simulink model "PIDp2"  (R2016b)
settings: Solver=FixedStepAuto  StartTime=0.0  StopTime=10.0  FixedStep=0.01  RelTol=1e-3
values from neighbouring files (symbols this model uses):
  den = [1 0.1313 1.109]    [UpdatedSimulinkValues-2.m]    (also in UpdatedSimulinkValuesalex1.m; part2a.m)
  Kd = G    [UpdatedSimulinkValues-2.m]    (also in UpdatedSimulinkValuesalex1.m; part2a.m = 0.1)
  Ki = G    [UpdatedSimulinkValues-2.m]    (also in UpdatedSimulinkValuesalex1.m; part2a.m = 0.1)
  Kp = G    [UpdatedSimulinkValues-2.m]    (also in UpdatedSimulinkValuesalex1.m; part2a.m = 0.1)
  num = [0.26*1.109*180/pi()]    [UpdatedSimulinkValues-2.m]    (also in UpdatedSimulinkValuesalex1.m; part2a.m)
settings Model: Creator=Akash  LastModifiedBy=Alex
settings SolverCC: MaxConsecutiveMinStep=2

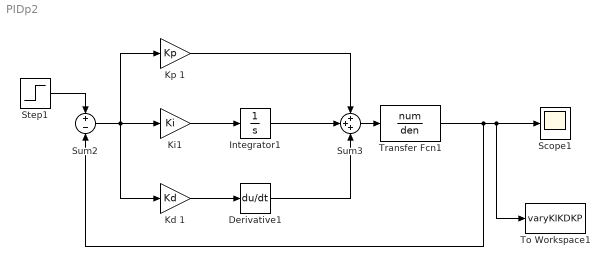
== system PIDp2 ==
  Derivative1 : Derivative
  Integrator1 : Integrator
  Kd 1 : Gain  Gain=Kd
  Ki1 : Gain  Gain=Ki
  Kp 1 : Gain  Gain=Kp
  Scope1 : Scope
  Step1 : Step  Time=0  SampleTime=0
  Sum2 : Sum  Inputs=+-
  Sum3 : Sum  Inputs=+++
  To Workspace1 : ToWorkspace  VariableName=varyKIKDKP  SaveFormat=Timeseries  SampleTime=-1
  Transfer Fcn1 : TransferFcn  Numerator=num  Denominator=den
  wires:
  Transfer Fcn1/1 -> Scope1/1, To Workspace1/1, Sum2/2
  Step1/1 -> Sum2/1
  Sum2/1 -> Kp 1/1, Kd 1/1, Ki1/1
  Ki1/1 -> Integrator1/1
  Integrator1/1 -> Sum3/2
  Kd 1/1 -> Derivative1/1
  Derivative1/1 -> Sum3/3
  Kp 1/1 -> Sum3/1
  Sum3/1 -> Transfer Fcn1/1
